simulink model "obsint_mdl"  (R2021b)
settings: Solver=ode1  StartTime=0.0  StopTime=20  FixedStep=0.01  MaxStep=0.1  MinStep=0.001  RelTol=1e-3
values from neighbouring files (symbols this model uses):
  A = A([2:end],[2:end])    [obsint_data.m]
  B = B([2:end],:)    [obsint_data.m]
  C = C(:,:)    [obsint_data.m]
  D = zeros(p,m)    [obsint_data.m]
  delta = 0.001    [obsint_data.m]    (also in outmodc_data.m)
  G = -inv(C*inv(A+B*F)*B)    [obsint_data.m]
  Gamma = diag([-10.0])    [obsint_data.m]
  pm = size(Cc,1)    [obsint_data.m]
  Ramp = 1000    [obsint_data.m]
  rho = 1    [obsint_data.m]    (also in outmodc_data.m)
  S = rpp(Ai,Bi,Eopt)    [obsint_data.m]
  Tc = Cc*inv(eye(n))    [obsint_data.m]
  z0 = zeros(1,n)    [obsint_data.m]
undefined symbols (not defined in the file or in its folder): F, L, Lam, Lr, Lrdot, m, n, P, Sr
libraries: simulink x1
settings Model: Creator=Witali  LastModifiedBy=w.schwamm
settings DataIOCC: SaveOutput=off  SaveTime=off  ReturnWorkspaceOutputs=off  StateSaveName=x  TimeSaveName=t  OutputSaveName=y

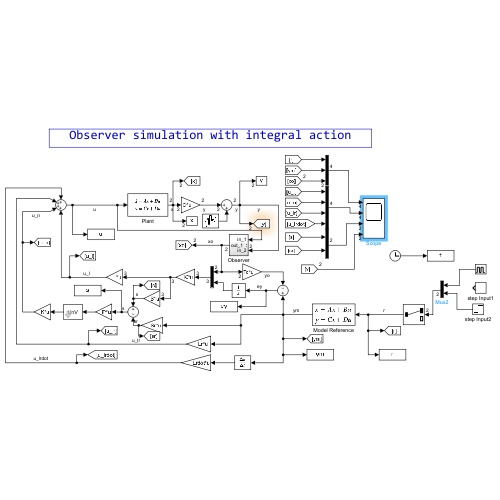
[thumbnail: Simulink's stored preview of the top-level diagram]
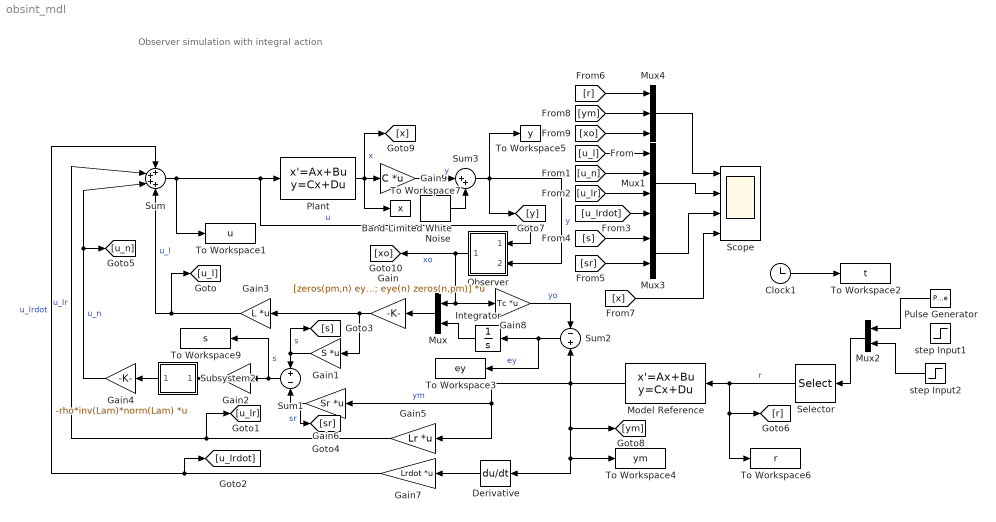
== system obsint_mdl ==
  note: Observer simulation with integral action
  Band-Limited White Noise : simulink/Sources/Band-Limited White Noise  Cov=[0.1]  Ts=0.01  seed=[23341]
  Clock1 : Clock
  Derivative : Derivative
  Gain : Gain  Gain=[zeros(pm,n) eye(pm); eye(n) zeros(n,pm)]  Multiplication=Matrix(K*u)
  Gain1 : Gain  Gain=S  Multiplication=Matrix(K*u)
  Gain2 : Gain  Gain=P  Multiplication=Matrix(K*u)
  Gain3 : Gain  Gain=L  Multiplication=Matrix(K*u)
  Gain4 : Gain  Gain=-rho*inv(Lam)*norm(Lam)  Multiplication=Matrix(K*u)
  Gain5 : Gain  Gain=Lr  Multiplication=Matrix(K*u)
  Gain6 : Gain  Gain=Sr  Multiplication=Matrix(K*u)
  Gain7 : Gain  Gain=Lrdot  Multiplication=Matrix(K*u)
  Gain8 : Gain  Gain=Tc  Multiplication=Matrix(K*u)
  Gain9 : Gain  Gain=C  Multiplication=Matrix(K*u)
  Integrator : Integrator
  Model Reference : StateSpace  A=Gamma  B=Gamma  C=-eye(pm)  D=zeros(pm,pm)  InitialCondition=0
  Mux : Mux  Inputs=2
  Mux1 : Mux
  Mux2 : Mux  Inputs=2
  Mux3 : Mux  Inputs=2
  Mux4 : Mux  Inputs=3
  Observer : Subsystem
  Plant : StateSpace  A=A  B=B  C=eye(n)  D=D  InitialCondition=0
  Pulse Generator : DiscretePulseGenerator  PulseType=Time based  Amplitude=Ramp  Period=10  PulseWidth=50
  Scope : Scope  NumInputPorts=4
  Selector : Selector  InputPortWidth=2  IndexOptions=Index vector (dialog)  Indices=[1:m]  OutputSizes=1
  Subsystem2 : Subsystem  mask{delta=1}
      mask prompts: delta "Unit vector delta:"
      mask Display: disp('UnV')
  Sum : Sum  Inputs=++++
  Sum1 : Sum  Inputs=+-
  Sum2 : Sum  Inputs=-+
  Sum3 : Sum  Inputs=|++
  To Workspace1 : ToWorkspace  VariableName=u  SaveFormat=Timeseries  SampleTime=-1
      settings: MaxDataPoints=1000000
  To Workspace2 : ToWorkspace  VariableName=t  SaveFormat=Timeseries  SampleTime=-1
      settings: MaxDataPoints=1000000
  To Workspace3 : ToWorkspace  VariableName=ey  SaveFormat=Timeseries  SampleTime=-1
      settings: MaxDataPoints=1000000
  To Workspace4 : ToWorkspace  VariableName=ym  SaveFormat=Timeseries  SampleTime=-1
      settings: MaxDataPoints=1000000
  To Workspace5 : ToWorkspace  VariableName=y  SaveFormat=Timeseries  SampleTime=-1
      settings: MaxDataPoints=1000000
  To Workspace6 : ToWorkspace  VariableName=r  SaveFormat=Timeseries  SampleTime=-1
      settings: MaxDataPoints=1000000
  To Workspace7 : ToWorkspace  VariableName=x  SaveFormat=Timeseries  SampleTime=-1
      settings: MaxDataPoints=1000000
  To Workspace9 : ToWorkspace  VariableName=s  SaveFormat=Timeseries  SampleTime=-1
      settings: MaxDataPoints=1000000
  step Input1 : Step  Time=Ramp  SampleTime=0
  step Input2 : Step  Time=0  After=0  SampleTime=0
  wires:
  Subsystem2/1(Out1) -> Gain4/1
  Gain2/1 -> Subsystem2/1(In1)
  Gain7/1 -> [u_lrdot], Sum/1  "u_lrdot"
  Sum/1 -> To Workspace1/1, Plant/1, Observer/1(in_1)  "u"
  Sum1/1 -> To Workspace9/1, Gain2/1  "s"
  Gain1/1 -> [s], Sum1/1  "s"
  Gain6/1 -> [sr], Sum1/2  "sr"
  Gain4/1 -> [u_n], Sum/3  "u_n"
  Gain3/1 -> [u_l], Sum/4  "u_l"
  Sum2/1 -> To Workspace3/1, Integrator/1  "ey"
  Derivative/1 -> Gain7/1
  Gain5/1 -> [u_lr], Sum/2  "u_lr"
  Gain/1 -> Gain3/1, Gain1/1
  Integrator/1 -> Mux/2
  Sum3/1 -> Observer/2(in_2), [y], To Workspace5/1  "y"
  Model Reference/1 -> Gain6/1, Gain5/1, [ym], To Workspace4/1, Derivative/1, Sum2/2  "ym"
  Clock1/1 -> To Workspace2/1
  Observer/1(out_1) -> Gain8/1, Mux/1, [xo]  "xo"
  Mux/1 -> Gain/1
  step Input2/1 -> Mux2/2
  [u_l] -> Mux1/1
  [u_n] -> Mux1/2
  [u_lr] -> Mux1/3
  [u_lrdot] -> Mux1/4
  Mux1/1 -> Scope/2
  [s] -> Mux3/1
  [sr] -> Mux3/2
  [r] -> Mux4/1
  Mux4/1 -> Scope/1
  Mux3/1 -> Scope/3
  Selector/1 -> To Workspace6/1, [r], Model Reference/1  "r"
  Mux2/1 -> Selector/1
  [xo] -> Mux4/3
  Plant/1 -> To Workspace7/1, [x], Gain9/1  "x"
  Gain8/1 -> Sum2/1  "yo"
  Pulse Generator/1 -> Mux2/1
  Gain9/1 -> Sum3/1  "y"
  Band-Limited White Noise/1 -> Sum3/2
  [ym] -> Mux4/2
  [x] -> Scope/4

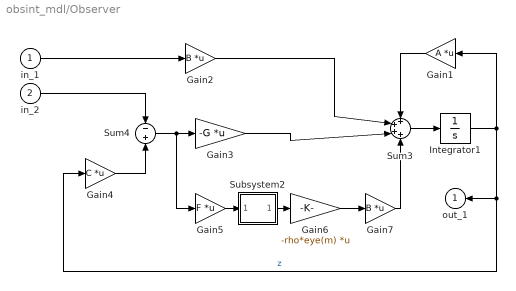
== system obsint_mdl/Observer ==
  in_1 : Inport
  in_2 : Inport  Port=2
  Gain1 : Gain  Gain=A  Multiplication=Matrix(K*u)
  Gain2 : Gain  Gain=B  Multiplication=Matrix(K*u)
  Gain3 : Gain  Gain=-G  Multiplication=Matrix(K*u)
  Gain4 : Gain  Gain=C  Multiplication=Matrix(K*u)
  Gain5 : Gain  Gain=F  Multiplication=Matrix(K*u)
  Gain6 : Gain  Gain=-rho*eye(m)  Multiplication=Matrix(K*u)
  Gain7 : Gain  Gain=B  Multiplication=Matrix(K*u)
  Integrator1 : Integrator  InitialCondition=z0
  Subsystem2 : Subsystem  mask{delta=delta}
      mask prompts: delta "Unit vector delta:"
      mask Display: disp('UnV')
  Sum3 : Sum  Inputs=++++
  Sum4 : Sum  Inputs=-+
  out_1 : Outport
  wires:
  Sum4/1 -> Gain5/1, Gain3/1
  Integrator1/1 -> Gain1/1, Gain4/1, out_1/1  "z"
  Gain4/1 -> Sum4/2
  Gain2/1 -> Sum3/2
  Gain6/1 -> Gain7/1
  Gain5/1 -> Subsystem2/1(In1)
  Subsystem2/1(Out1) -> Gain6/1
  Gain7/1 -> Sum3/4
  Gain3/1 -> Sum3/3
  Gain1/1 -> Sum3/1
  Sum3/1 -> Integrator1/1
  in_1/1 -> Gain2/1
  in_2/1 -> Sum4/1

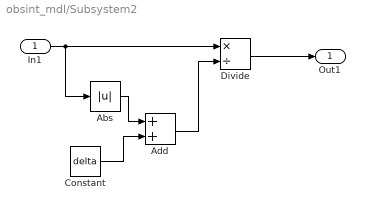
== system obsint_mdl/Subsystem2 ==
  In1 : Inport
  Abs : Abs
  Add : Sum
  Constant : Constant  Value=delta  SampleTime=-1
  Divide : Product  Inputs=*/
  Out1 : Outport
  wires:
  Constant/1 -> Add/2
  Add/1 -> Divide/2
  Abs/1 -> Add/1
  Divide/1 -> Out1/1
  In1/1 -> Divide/1, Abs/1

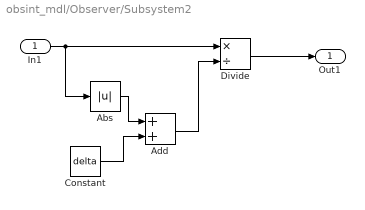
== system obsint_mdl/Observer/Subsystem2 ==
  In1 : Inport
  Abs : Abs
  Add : Sum
  Constant : Constant  Value=delta  SampleTime=-1
  Divide : Product  Inputs=*/
  Out1 : Outport
  wires:
  Constant/1 -> Add/2
  Add/1 -> Divide/2
  Abs/1 -> Add/1
  Divide/1 -> Out1/1
  In1/1 -> Divide/1, Abs/1
